simulink model "positionerrors"  (R2019b)
settings: Solver=VariableStepAuto  StartTime=0.0  StopTime=10.0  RelTol=1e-3
settings Model: Creator=Pablo  LastModifiedBy=Pablo

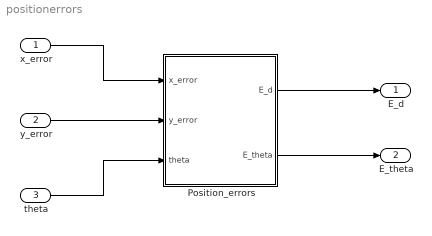
== system positionerrors ==
  x_error : Inport
  y_error : Inport  Port=2
  theta : Inport  Port=3
  Position_errors : Subsystem
  E_d : Outport
  E_theta : Outport  Port=2
  wires:
  x_error/1 -> Position_errors/1(x_error)
  y_error/1 -> Position_errors/2(y_error)
  theta/1 -> Position_errors/3(theta)
  Position_errors/1(E_d) -> E_d/1
  Position_errors/2(E_theta) -> E_theta/1

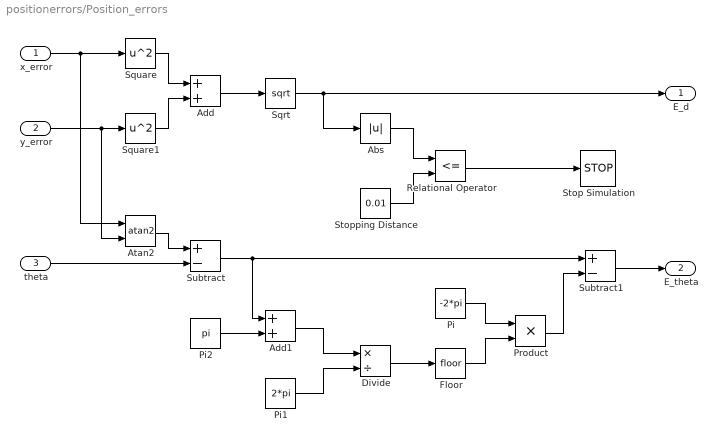
== system positionerrors/Position_errors ==
  x_error : Inport
  y_error : Inport  Port=2
  theta : Inport  Port=3
  Abs : Abs
  Add : Sum
  Add1 : Sum
  Atan2 : Trigonometry  Operator=atan2
  Divide : Product  Inputs=*/
  Floor : Rounding
  Pi : Constant  Value=-2*pi  OutDataTypeStr=Inherit: Inherit via back propagation
  Pi1 : Constant  Value=2*pi  OutDataTypeStr=Inherit: Inherit via back propagation
  Pi2 : Constant  Value=pi  OutDataTypeStr=Inherit: Inherit via back propagation
  Product : Product
  Relational Operator : RelationalOperator  Operator=<=  OutDataTypeStr=boolean  RndMeth=Simplest
  Sqrt : Sqrt  SaturateOnIntegerOverflow=on
  Square : Math  Operator=square  SignedPower=off  SaturateOnIntegerOverflow=on
  Square1 : Math  Operator=square  SignedPower=off  SaturateOnIntegerOverflow=on
  "Stop Simulation " : Stop
  Stopping Distance : Constant  Value=0.01
  Subtract : Sum  Inputs=+-
  Subtract1 : Sum  Inputs=+-
  E_d : Outport
  E_theta : Outport  Port=2
  wires:
  y_error/1 -> Atan2/2, Square1/1
  x_error/1 -> Atan2/1, Square/1
  Sqrt/1 -> E_d/1, Abs/1
  Relational Operator/1 -> "Stop Simulation "/1
  Add1/1 -> Divide/1
  Product/1 -> Subtract1/2
  Square/1 -> Add/1
  theta/1 -> Subtract/2
  Pi1/1 -> Divide/2
  Square1/1 -> Add/2
  Add/1 -> Sqrt/1
  Atan2/1 -> Subtract/1
  Subtract/1 -> Subtract1/1, Add1/1
  Divide/1 -> Floor/1
  Pi/1 -> Product/1
  Subtract1/1 -> E_theta/1
  Abs/1 -> Relational Operator/1
  Floor/1 -> Product/2
  Stopping Distance/1 -> Relational Operator/2
  Pi2/1 -> Add1/2
